simulink model "model5_1"  (R2024b)
settings: Solver=VariableStepAuto  StartTime=0.0  StopTime=20  RelTol=1e-3
values from neighbouring files (symbols this model uses):
  R = (1 - 2 * c * z^(-1) + z^(-2)) / (s * z^(-1)) * R0    [domaci5_2_d.m]
  S = tf(double([sol.s3, sol.s2, sol.s1, sol.s0]), 1, Ts)    [domaci5_2_d.m]
  T = 1 / dcgain(minreal(1 / R * feedback(Gpd, S / R), 1e-2))    [domaci5_2_d.m]
settings Model: Creator=neso  LastModifiedBy=neso

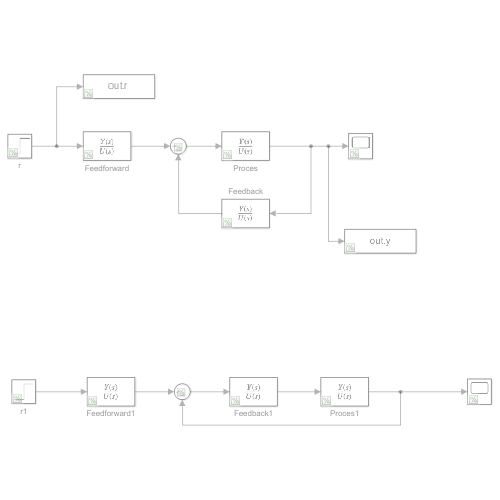
[thumbnail: Simulink's stored preview of the top-level diagram]
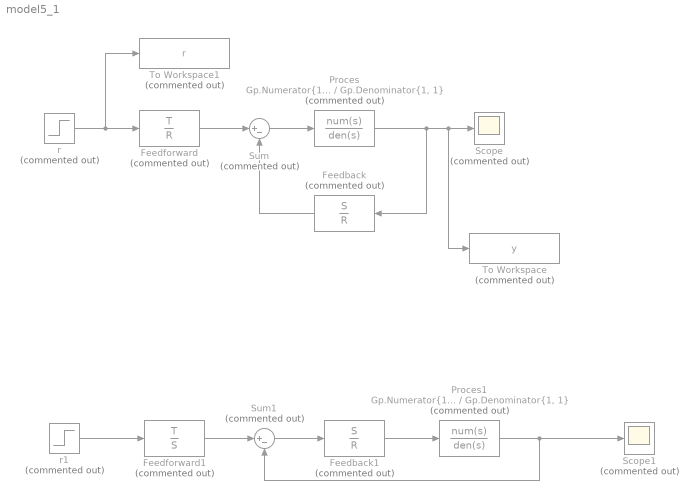
== system model5_1 ==
  Feedback : TransferFcn  Commented=on  Numerator=S  Denominator=R
  Feedback1 : TransferFcn  Commented=on  Numerator=S  Denominator=R
  Feedforward : TransferFcn  Commented=on  Numerator=T  Denominator=R
  Feedforward1 : TransferFcn  Commented=on  Numerator=T  Denominator=S
  Proces : TransferFcn  Commented=on  Numerator=Gp.Numerator{1, 1}  Denominator=Gp.Denominator{1, 1}
  Proces1 : TransferFcn  Commented=on  Numerator=Gp.Numerator{1, 1}  Denominator=Gp.Denominator{1, 1}
  Scope : Scope  Commented=on
  Scope1 : Scope  Commented=on
  Sum : Sum  Commented=on  Inputs=|+-
  Sum1 : Sum  Commented=on  Inputs=|+-
  To Workspace : ToWorkspace  Commented=on  VariableName=y  SaveFormat=Timeseries  SampleTime=-1
  To Workspace1 : ToWorkspace  Commented=on  VariableName=r  SaveFormat=Timeseries  SampleTime=-1
  r : Step  Commented=on  Time=0  After=5  SampleTime=0
  r1 : Step  Commented=on  Time=0  After=5  SampleTime=0
  wires:
  Feedforward/1 -> Sum/1
  Sum/1 -> Proces/1
  Feedback/1 -> Sum/2
  r/1 -> To Workspace1/1, Feedforward/1
  Proces/1 -> To Workspace/1, Scope/1, Feedback/1
  Feedforward1/1 -> Sum1/1
  r1/1 -> Feedforward1/1
  Proces1/1 -> Scope1/1, Sum1/2
  Sum1/1 -> Feedback1/1
  Feedback1/1 -> Proces1/1
